simulink model "dspwvtrnsmx"  (Simulink 5.0)
settings: Solver=FixedStepDiscrete  SolverMode=SingleTasking  StartTime=0.0  StopTime=1000  RelTol=1e-3
PreLoadFcn:
  | load dspwlets;
values from neighbouring files (symbols this model uses):
  ts = [-1 0]    [lmsxy.m]    (also in sdspwwvdisp.m = get_param(blk,'CompiledSampleTime'))
undefined symbols (not defined in the file or in its folder): hir, lor
libraries: dspmlti4 x4, dspsrcs4 x3, dspsigops x3
settings Model: Creator=don  LastModifiedBy=mkhan  ExtModeTrigMode=oneshot  ExtModeArmWhenConnect=off  SaveTime=off  SaveOutput=off  LimitDataPoints=off  IntegerOverflowMsg=none  BlockReductionOpt=off  BooleanDataType=off  ZeroCrossControl=UseLocalSettings  TargetHWChar=2  TargetHWWordLengths=8,16,32,32  RTWMathFcnLibMatFile=iso_c_tmw.mat  RTWOptions="-aEnforceIntegerDowncast=1 -aFoldNonRolledExpr=1 -aInlineInvariantSignals=1 -aInlineParameters=0 -aLocalBlockOutputs=1 -aRollThreshold=2 -aRTWVerbose=1 -aForceParamTrailComments=0 -aGenerateComments=1 -aIgnoreCustomStorageClasses=1 -aIncHierarchyInIds=0 -aMaxRTWIdLen=31 -aShowEliminatedStatements=1 -aReadOnly=0 -aTargetFcnLib=\"iso_c_tmw.mat\" -aIncDataTypeInIds=0 -aPrefixModelToSubsysFcnNames=1 -aInlinedPrmAccess=\"Literals\" -aGenerateFullHeader=1 -aIsPILTarget=0 -aGenerateReport=0 -aLogVarNameModifier=\"rt_\" -aExtMode=0 -aExtModeStaticAlloc=0 -aExtModeTesting=0 -aExtModeStaticAllocSize=1000000 -aExtModeTransport=0  -aCGOptsFile=\"dsp_cgopts\""

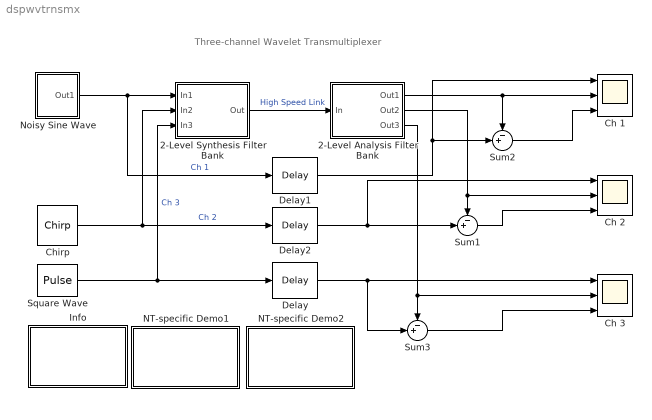
== system dspwvtrnsmx ==
  note: Three-channel Wavelet Transmultiplexer
  2-Level Analysis Filter Bank : Subsystem
  2-Level Synthesis Filter Bank : Subsystem
  Ch 1 : Scope  NumInputPorts=3
      settings: TimeRange=1000  YMin=-2~-2~-5e-011  YMax=2~2~5e-011
  Ch 2 : Scope  NumInputPorts=3
      settings: TimeRange=1000  YMin=-1~-1~-5e-011  YMax=1~1~5e-011
  Ch 3 : Scope  NumInputPorts=3
      settings: TimeRange=1000  YMin=0~0~-5e-011  YMax=1.2~1.2~5e-011  SaveName=ScopeData2
  Chirp : dspsrcs4/Chirp  sweep=Swept cosine  mode=Bidirectional  f0=1/5000  f1=1/50  t1=1000  Tsweep=1000  phase=0  Ts=ts  spf=1  datatype=Double
  Delay : dspsigops/Delay  dly_unit=Samples  delay=6  ic_detail=on  dif_ic_for_ch=off  dif_ic_for_dly=off  ic=0  reset_popup=None
  Delay1 : dspsigops/Delay  dly_unit=Samples  delay=4  ic_detail=on  dif_ic_for_ch=off  dif_ic_for_dly=off  ic=0  reset_popup=None
  Delay2 : dspsigops/Delay  dly_unit=Samples  delay=6  ic_detail=on  dif_ic_for_ch=off  dif_ic_for_dly=off  ic=0  reset_popup=None
  Info : Subsystem
      mask Type: Frame-Based Simulation Info
      mask Display: disp('Info')
  NT-specific Demo1 : Subsystem
      settings: OpenFcn=dspwvtrnsmxf
      mask Type: Frame-Based Demo
      mask Display: disp('Frame-Based\nDemo')
  NT-specific Demo2 : Subsystem
      settings: OpenFcn=dspwvtrnsmxfp
      mask Type: Fixed-Point Demo
      mask Display: disp('Fixed-Point\nDemo')
  Noisy Sine Wave : Subsystem  mask(Noisy Sine Wave){}
      mask init:
      | dx=pi/5;
      | x=(0:dx:2*pi)';
      | y=sin(x);
      | [x,y]=stairs(x,y);
      | 
      | % Axes:
      | x=[x;NaN;0; 0;NaN;0;2*pi];
      | y=[y;NaN;1;-1;NaN;0;0];
      mask Display: plot(x,y)
  Square Wave : DiscretePulseGenerator  Period=125  PulseWidth=50  SampleTime=ts  VectorParams1D=off
  Sum1 : Sum  Inputs=-+|  SaturateOnIntegerOverflow=on  InputSameDT=on
  Sum2 : Sum  Inputs=-+|  SaturateOnIntegerOverflow=on  InputSameDT=on
  Sum3 : Sum  Inputs=-+|  SaturateOnIntegerOverflow=on  InputSameDT=on
  wires:
  Chirp/1 -> 2-Level Synthesis Filter Bank/2(In2), Delay2/1  "Ch 2"
  2-Level Analysis Filter Bank/2(Out2) -> Ch 2/2, Sum1/1
  2-Level Analysis Filter Bank/1(Out1) -> Ch 1/2, Sum2/1
  2-Level Synthesis Filter Bank/1(Out) -> 2-Level Analysis Filter Bank/1(In)  "High Speed Link"
  Noisy Sine Wave/1(Out1) -> 2-Level Synthesis Filter Bank/1(In1), Delay1/1  "Ch 1"
  Delay2/1 -> Sum1/2, Ch 2/1
  Delay1/1 -> Ch 1/1, Sum2/2
  Square Wave/1 -> 2-Level Synthesis Filter Bank/3(In3), Delay/1  "Ch 3"
  2-Level Analysis Filter Bank/3(Out3) -> Sum3/1, Ch 3/2
  Sum2/1 -> Ch 1/3
  Sum1/1 -> Ch 2/3
  Sum3/1 -> Ch 3/3
  Delay/1 -> Ch 3/1, Sum3/2

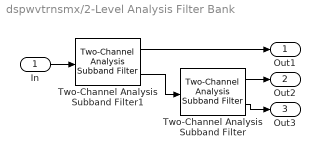
== system dspwvtrnsmx/2-Level Analysis Filter Bank ==
  In : Inport
  Two-Channel Analysis Subband Filter : dspmlti4/Two-Channel Analysis Subband Filter  lpf=lod  hpf=hid  framing=Maintain input frame size
  Two-Channel Analysis Subband Filter1 : dspmlti4/Two-Channel Analysis Subband Filter  lpf=lod  hpf=hid  framing=Maintain input frame size
  Out1 : Outport
  Out2 : Outport  Port=2
  Out3 : Outport  Port=3
  wires:
  In/1 -> Two-Channel Analysis Subband Filter1/1
  Two-Channel Analysis Subband Filter1/1 -> Out1/1
  Two-Channel Analysis Subband Filter1/2 -> Two-Channel Analysis Subband Filter/1
  Two-Channel Analysis Subband Filter/1 -> Out2/1
  Two-Channel Analysis Subband Filter/2 -> Out3/1

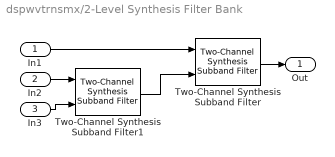
== system dspwvtrnsmx/2-Level Synthesis Filter Bank ==
  In1 : Inport
  In2 : Inport  Port=2
  In3 : Inport  Port=3
  Two-Channel Synthesis Subband Filter : dspmlti4/Two-Channel Synthesis Subband Filter  lpf=[0 lor]  hpf=[0 hir]  framing=Maintain input frame size
  Two-Channel Synthesis Subband Filter1 : dspmlti4/Two-Channel Synthesis Subband Filter  lpf=[0 lor]  hpf=[0 hir]  framing=Maintain input frame size
  Out : Outport
  wires:
  In3/1 -> Two-Channel Synthesis Subband Filter1/2
  In2/1 -> Two-Channel Synthesis Subband Filter1/1
  Two-Channel Synthesis Subband Filter/1 -> Out/1
  In1/1 -> Two-Channel Synthesis Subband Filter/1
  Two-Channel Synthesis Subband Filter1/1 -> Two-Channel Synthesis Subband Filter/2

== system dspwvtrnsmx/Info ==
  note: Demonstration of a Wavelet Transmultiplexer (WTM)
      |
      | The wavelet transmultiplexer (WTM) provides
      | an interesting example of the perfect
      | reconstruction property of the DWT.
      |
      | This WTM combines three source signals for transmission
      | over a single link, then separates the three signals at the
      | receiving end of the channel.  The waveforms plotted in
      | each of the scope windows demonstrate the ability of wavelets
      | to provide perfect reconstruction of each of the three
      | independent signals, transmitted over a single communications
      | link.  The error trace is displayed with an expanded vertical
      | scale to demonstrate the absence of signal corruption.
      | This model demonstrates a three-channel transmultiplexer,
      | but the method can be extended to an arbitrary number of
      | channels.  Note that the total data rate is limited
      | by the Nyquist rate of the high-speed data link.
      |
      | The operation of a WTM is analogous to a frequency-domain
      | multiplexer (FDM) in several respects.  In an FDM, baseband
      | input signals are filtered and modulated into adjacent frequency
      | bands, summed together, then transmitted over a single link.
      | On the receiving end, the transmitted signal is filtered to separate
      | adjacent frequency channels, and the signals are demodulated
      | back to baseband.  The filters also must strongly attenuate the
      | adjacent signal to provide a sharp transition from the
      | filter passband to its stopband.  This process limits the
      | amount of crosstalk (signal leakage) from one frequency band
      | to the next.  In addition, often FDM employs
      | an unused frequency band between the three modulated
      | frequency bands (known as a guard band) to relax
      | the requirements on the FDM filters.
      |
      | In a WTM, the filtering performed by the synthesis
      | and analysis wavelet filters is analogous to the
      | filtering steps in the FDM, and the interpolation in the
      | IDWT is equivalent to frequency modulation.  From a
      | frequency domain perspective, the wavelet filters
      | are fairly poor spectral filters (as compared to the filters
      | required by a FDM implementation), exhibiting slow transitions
      | from passband to stopband, and providing significant
      | distortion in their response.  What makes the WTM special
      | is that the analysis and synthesis filters together
      | completely cancel the filter distortions and signal aliasing,
      | producing perfect reconstruction of the input signals
      | and thus perfect extraction of the multiplexed inputs.
      | Ideal spectral efficiency can be achieved, since no guard
      | band is required.  Practical limitations in the implementation
      | of channel filters create out-of-band leakage and distortion.
      | In the conventional FDM approach, each channel within the
      | same communications system requires its own filter and is
      | susceptible to crosstalk from neighboring channels.  With the
      | WTM method, only a single bandpass filter is required
      | for the entire communications channel, while channel-to-channel
      | interference is eliminated.
      |
      | Note that a noisy link can cause imperfect reconstruction of the
      | input signals, and the effects of channel noise and other impairments
      | in the recovered signals can differ in FDM and WTM.  This can be
      | modeled, for example, by adding a noise source to the high speed link.

== system dspwvtrnsmx/NT-specific Demo1 ==

== system dspwvtrnsmx/NT-specific Demo2 ==

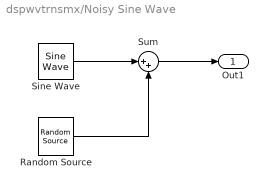
== system dspwvtrnsmx/Noisy Sine Wave ==
  Random Source : dspsrcs4/Random Source  SrcType=Gaussian  Min=0  Max=1  Mean=0  Var=0.2  RepMode=Specify seed  Seed=1  Inherit=off  SampMode=Discrete  SampTime=ts/2  SampFrame=1  OutComplex=Real
  Sine Wave : dspsrcs4/Sine Wave  Amplitude=1  Frequency=1/68  Phase=0  SampleMode=Discrete  OutComplex=Real  CompMethod=Trigonometric fcn  TableSize=Speed  SampleTime=ts/2  SamplesPerFrame=1  dType=Double  ResetState=Restart at time zero
  Sum : Sum  Inputs=|++  SaturateOnIntegerOverflow=on  InputSameDT=on
  Out1 : Outport
  wires:
  Sum/1 -> Out1/1
  Sine Wave/1 -> Sum/1
  Random Source/1 -> Sum/2
